simulink model "telemedicine_screening_model"  (R2026a)
settings: Solver=ode45  StopTime=28800
settings Model: Creator=user  LastModifiedBy=user
settings DataIOCC: OutputSaveName=simout

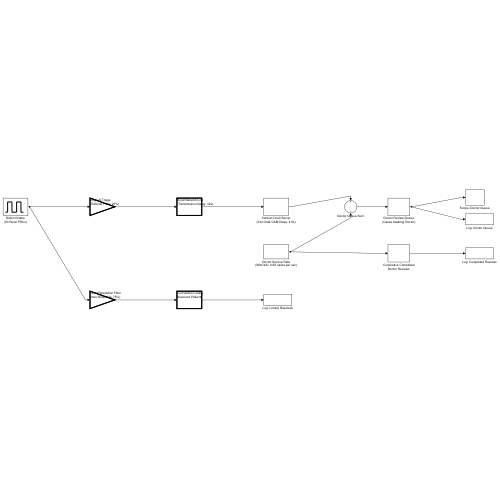
[thumbnail: Simulink's stored preview of the top-level diagram]
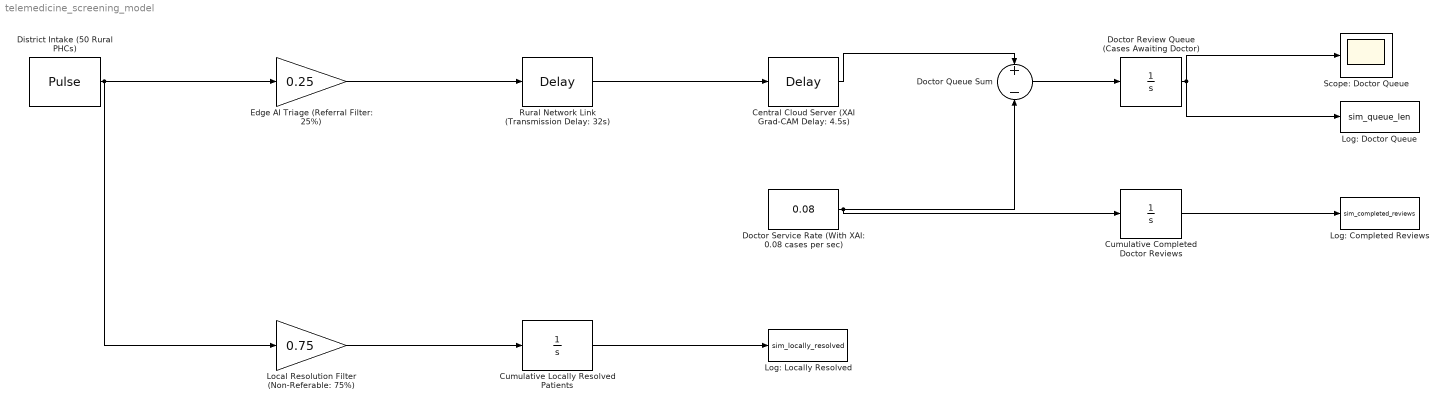
== system telemedicine_screening_model ==
  Central Cloud Server (XAI Grad-CAM Delay: 4.5s) : TransportDelay  DelayTime=4.5
  Cumulative Completed Doctor Reviews : Integrator
  Cumulative Locally Resolved Patients : Integrator
  District Intake (50 Rural PHCs) : DiscretePulseGenerator  PulseType=Time based  Period=54  PulseWidth=50
  Doctor Queue Sum : Sum  Inputs=+-
  Doctor Review Queue (Cases Awaiting Doctor) : Integrator  LimitOutput=on  LowerSaturationLimit=0
  Doctor Service Rate (With XAI: 0.08 cases per sec) : Constant  Value=0.08
  Edge AI Triage (Referral Filter: 25%) : Gain  Gain=0.25
  Local Resolution Filter (Non-Referable: 75%) : Gain  Gain=0.75
  Log: Completed Reviews : ToWorkspace  VariableName=sim_completed_reviews  SampleTime=-1
  Log: Doctor Queue : ToWorkspace  VariableName=sim_queue_len  SampleTime=-1
  Log: Locally Resolved : ToWorkspace  VariableName=sim_locally_resolved  SampleTime=-1
  Rural Network Link (Transmission Delay: 32s) : TransportDelay  DelayTime=32.0
  Scope: Doctor Queue : Scope
  wires:
  District Intake (50 Rural PHCs)/1 -> Edge AI Triage (Referral Filter: 25%)/1, Local Resolution Filter (Non-Referable: 75%)/1
  Edge AI Triage (Referral Filter: 25%)/1 -> Rural Network Link (Transmission Delay: 32s)/1
  Rural Network Link (Transmission Delay: 32s)/1 -> Central Cloud Server (XAI Grad-CAM Delay: 4.5s)/1
  Central Cloud Server (XAI Grad-CAM Delay: 4.5s)/1 -> Doctor Queue Sum/1
  Doctor Queue Sum/1 -> Doctor Review Queue (Cases Awaiting Doctor)/1
  Doctor Review Queue (Cases Awaiting Doctor)/1 -> Scope: Doctor Queue/1, Log: Doctor Queue/1
  Doctor Service Rate (With XAI: 0.08 cases per sec)/1 -> Doctor Queue Sum/2, Cumulative Completed Doctor Reviews/1
  Cumulative Completed Doctor Reviews/1 -> Log: Completed Reviews/1
  Local Resolution Filter (Non-Referable: 75%)/1 -> Cumulative Locally Resolved Patients/1
  Cumulative Locally Resolved Patients/1 -> Log: Locally Resolved/1
